simulink model "FOC_BLDC_HIL"  (R2021a)
settings: Solver=FixedStepDiscrete  StartTime=0.0  StopTime=2  RelTol=1e-3  EnableMultiTasking=on
undefined symbols (not defined in the file): DiscIntNeverNeededParam, Init_angle, J, Kawspeed, Ke, Kspeed, Lsx, Lsy, negVid, negVTm, oversampling, p, posVid, posVTm, Psim, Rs, T_load, Ts, ts_FPGA_clk, ts_FPGA_mdl, Ts_svpwm, Tsp, Vdc, Viq, VTm
libraries: simulink x93, hdlsllib x23, slrealtimeloglib x3
(part 1 of 4)
settings Model: SimulationMode=accelerator  Creator=jatin  LastModifiedBy=jatin
settings SolverCC: AutoInsertRateTranBlk=on
settings DataIOCC: SaveOutput=off  SignalLogging=off  DSMLogging=off  SaveTime=off  ReturnWorkspaceOutputs=off
settings OptimizationCC: BlockReduction=off  ConditionallyExecuteInputs=off  DefaultParameterBehavior=Inlined
settings DebuggingCC: AlgebraicLoopMsg=error  SingleTaskRateTransMsg=error  ParameterPrecisionLossMsg=none
settings HardwareCC: ProdBitPerPointer=32  ProdBitPerSizeT=32  ProdBitPerPtrDiffT=32  ProdLargestAtomicFloat=None  ProdIntDivRoundTo=Undefined  ProdEndianess=Unspecified  ProdWordSize=32  ProdHWDeviceType=ASIC/FPGA->ASIC/FPGA  TargetBitPerPointer=64  TargetBitPerSizeT=64  TargetBitPerPtrDiffT=64  TargetLongLongMode=on  TargetIntDivRoundTo=Zero  TargetEndianess=LittleEndian  TargetWordSize=64  TargetHWDeviceType=Custom Processor->MATLAB Host Computer  ProdEqTarget=off

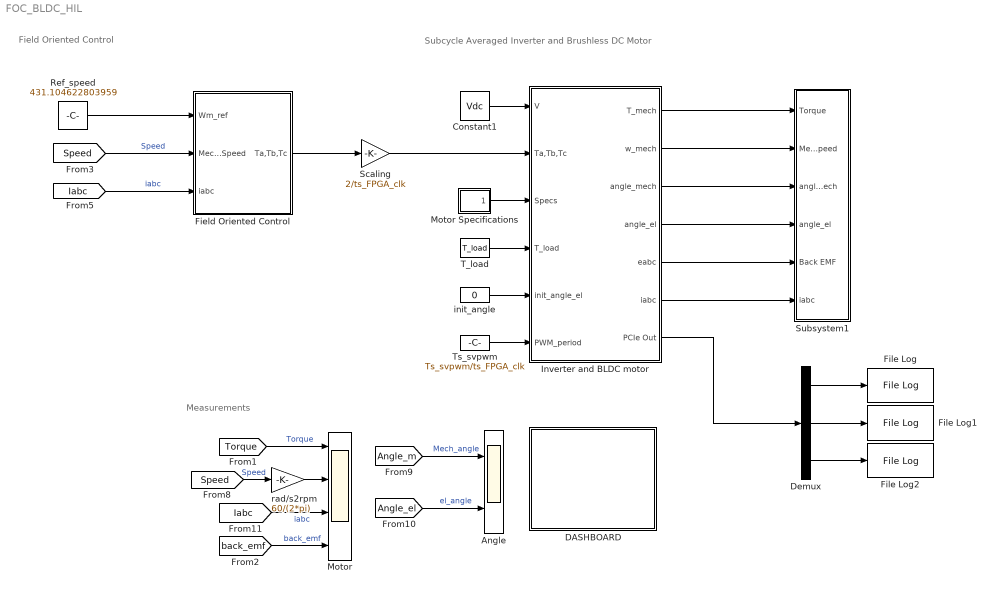
== system FOC_BLDC_HIL ==
  note: Subcycle Averaged Inverter and Brushless DC Motor
  note: Measurements
  note: Field Oriented Control
  Angle : Scope  NumInputPorts=2
  Constant1 : Constant  Value=Vdc  OutDataTypeStr=single  SampleTime=Ts
  DASHBOARD : Subsystem
  Demux : Demux  Outputs=3
  Field Oriented Control : Subsystem
  File Log : slrealtimeloglib/File Log  decimation=1
      settings: SourceProductBaseCode=XP
  File Log1 : slrealtimeloglib/File Log  decimation=1
      settings: SourceProductBaseCode=XP
  File Log2 : slrealtimeloglib/File Log  decimation=1
      settings: SourceProductBaseCode=XP
  Inverter and BLDC motor : Subsystem
  Motor : Scope  NumInputPorts=4
  Motor Specifications : Subsystem
  Ref_speed : Constant  Value=431.104622803959  OutDataTypeStr=single  SampleTime=Tsp
  Scaling : Gain  Gain=2/ts_FPGA_clk  OutDataTypeStr=int32
  Subsystem1 : Subsystem
  T_load : Constant  Value=T_load  OutDataTypeStr=single  SampleTime=Ts
  Ts_svpwm : Constant  Value=Ts_svpwm/ts_FPGA_clk  OutDataTypeStr=uint32  SampleTime=Ts
  init_angle : Constant  Value=0  OutDataTypeStr=single  SampleTime=Ts
  rad/s2rpm : Gain  Gain=60/(2*pi)
  wires:
  [Speed] -> Field Oriented Control/2(Mech_Speed)  "Speed"
  [Iabc] -> Motor/3  "iabc"
  [Angle_m] -> Angle/1  "Mech_angle"
  [Speed] -> rad/s2rpm/1  "Speed"
  [Torque] -> Motor/1  "Torque"
  [Angle_el] -> Angle/2  "el_angle"
  [Iabc] -> Field Oriented Control/3(iabc)  "iabc"
  Constant1/1 -> Inverter and BLDC motor/1(V)
  [back_emf] -> Motor/4  "back_emf"
  Motor Specifications/1(Specs) -> Inverter and BLDC motor/3(Specs)
  T_load/1 -> Inverter and BLDC motor/4(T_load)
  Inverter and BLDC motor/1(T_mech) -> Subsystem1/1(Torque)
  Inverter and BLDC motor/2(w_mech) -> Subsystem1/2(Mech_Speed)
  Inverter and BLDC motor/3(angle_mech) -> Subsystem1/3(angle_mech)
  Inverter and BLDC motor/4(angle_el) -> Subsystem1/4(angle_el)
  Inverter and BLDC motor/5(eabc) -> Subsystem1/5(Back EMF)
  Inverter and BLDC motor/6(iabc) -> Subsystem1/6(iabc)
  init_angle/1 -> Inverter and BLDC motor/5(init_angle_el)
  Ts_svpwm/1 -> Inverter and BLDC motor/6(PWM_period)
  Field Oriented Control/1(Ta,Tb,Tc) -> Scaling/1
  Scaling/1 -> Inverter and BLDC motor/2(Ta,Tb,Tc)
  rad/s2rpm/1 -> Motor/2
  Ref_speed/1 -> Field Oriented Control/1(Wm_ref)
  Demux/3 -> File Log2/1
  Demux/1 -> File Log/1
  Demux/2 -> File Log1/1
  Inverter and BLDC motor/7(PCIe Out) -> Demux/1
